simulink model "Part1_LQ"  (R2021a)
settings: Solver=ode45  StartTime=0.0  StopTime=10  RelTol=1e-3  EnableMultiTasking=on
values from neighbouring files (symbols this model uses):
  A = [0 1; -K/m -D/m]    [Part1.m]    (also in Part2.m = [zeros(2) eye(2))
  B = [0 ; 1]    [Part1.m]    (also in Part2.m = [zeros(2,1))
  Bp = [0 ; 1 ]    [Part1.m]    (also in Part2.m = [zeros(2,1))
  C = [1 0]    [Part1.m]    (also in Part2.m = [1 0 0 0])
  K_LQ = lqr(sys, Q, r^2)    [Part2.m]
  M = -inv(C*inv(A-B*K_LQ)*B)    [Part1.m]    (also in Part2.m)
  N = -inv(C*inv(A-B*K_LQ)*B)*(C*inv(A-B*K_LQ)*Bp)    [Part1.m]
settings Model: Creator=Tebbani  LastModifiedBy=Sihem Tebbani
settings SolverCC: AlgebraicLoopSolver=TrustRegion
settings DataIOCC: LimitDataPoints=on  SaveFormat=Array  ReturnWorkspaceOutputs=off
settings OptimizationCC: LifeSpan=inf
settings DebuggingCC: SolverPrmCheckMsg=warning  SFUnexpectedBacktrackingDiag=warning  SFNoUnconditionalDefaultTransitionDiag=warning  SFExecutionAtInitializationDiag=none  SFMachineParentedDataDiag=warning  ArithmeticOperatorsInVariantConditions=warning
settings HardwareCC: ProdBitPerPointer=32  ProdBitPerSizeT=32  ProdBitPerPtrDiffT=32  ProdLargestAtomicFloat=None  ProdIntDivRoundTo=Undefined  ProdEndianess=Unspecified  ProdWordSize=32  ProdHWDeviceType=32-bit Generic
settings ModelReferenceCC: PropagateSignalLabelsOutOfModel=off
settings SFSimCC: SimUseLocalCustomCode=off  CustomCodeUndefinedFunction=UseInterfaceOnly
settings RTWCC: RTWUseLocalCustomCode=off
settings CodeAppCC: StateflowObjectComments=on
settings GRTTargetCC: TargetLangStandard=C89/C90 (ANSI)
settings ConfigComp: CovMetricSettings=dw  CovSaveCumulativeToWorkspaceVar=on  CovSaveSingleToWorkspaceVar=on  CovExternalEMLEnable=off  CovSFcnEnable=off

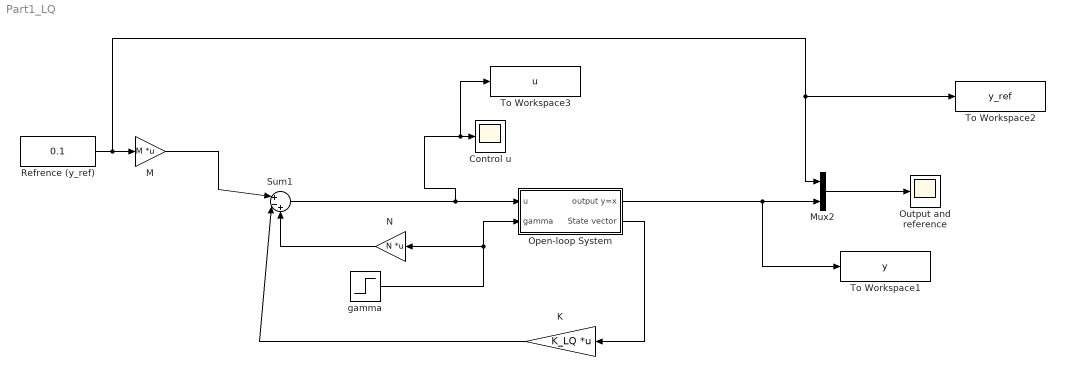
== system Part1_LQ ==
  Control u : Scope
  K : Gain  Gain=K_LQ  Multiplication=Matrix(K*u) (u vector)
  M : Gain  Gain=M  Multiplication=Matrix(K*u) (u vector)
  Mux2 : Mux  Inputs=2
  N : Gain  Gain=N  Multiplication=Matrix(K*u) (u vector)
  Open-loop System : Subsystem
  Output and reference : Scope
  Refrence (y_ref) : Constant  Value=0.1
  Sum1 : Sum  Inputs=|+-+
  To Workspace1 : ToWorkspace  VariableName=y  SaveFormat=Structure With Time  SampleTime=-1
  To Workspace2 : ToWorkspace  VariableName=y_ref  SaveFormat=Structure With Time  SampleTime=-1
  To Workspace3 : ToWorkspace  VariableName=u  SaveFormat=Structure With Time  SampleTime=-1
  gamma : Step  Time=5  SampleTime=0
  wires:
  Open-loop System/1(output y=x) -> To Workspace1/1, Mux2/2
  Mux2/1 -> Output and reference/1
  Open-loop System/2(State vector) -> K/1
  K/1 -> Sum1/2
  N/1 -> Sum1/3
  Sum1/1 -> To Workspace3/1, Control u/1, Open-loop System/1(u)
  Refrence (y_ref)/1 -> To Workspace2/1, Mux2/1, M/1
  M/1 -> Sum1/1
  gamma/1 -> N/1, Open-loop System/2(gamma)

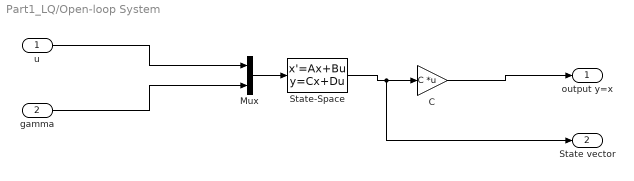
== system Part1_LQ/Open-loop System ==
  u : Inport
  gamma : Inport  Port=2
  C : Gain  Gain=C  Multiplication=Matrix(K*u) (u vector)
  Mux : Mux  Inputs=2
  State-Space : StateSpace  A=A  B=[B Bp]  C=eye(2)  D=zeros(2)  InitialCondition=[0. 0]
  output y=x : Outport
  State vector : Outport  Port=2
  wires:
  Mux/1 -> State-Space/1
  gamma/1 -> Mux/2
  u/1 -> Mux/1
  State-Space/1 -> State vector/1, C/1
  C/1 -> output y=x/1
